simulink model "stateflow_reuseVariable"  (R2016b)
settings: Solver=VariableStepAuto  StartTime=0.0  StopTime=10.0  RelTol=1e-3  EnableMultiTasking=on
settings Model: Creator=amyyang  LastModifiedBy=amyyang
settings DataIOCC: LimitDataPoints=on
settings OptimizationCC: LifeSpan=inf
settings DebuggingCC: AllowSymbolicDim=off  SFUnexpectedBacktrackingDiag=warning  SFNoUnconditionalDefaultTransitionDiag=warning  SFExecutionAtInitializationDiag=none
settings ModelReferenceCC: PropagateSignalLabelsOutOfModel=off
settings GRTTargetCC: TargetLangStandard=C89/C90 (ANSI)
settings ConfigComp: CovMetricSettings=dw  CovHtmlReporting=on  CovSaveCumulativeToWorkspaceVar=on  CovSaveSingleToWorkspaceVar=on  CovExternalEMLEnable=off

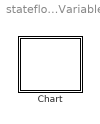
== system stateflow_reuseVariable ==
  Chart : Stateflow chart  TreatAsAtomicUnit=on

== stateflow chart stateflow_reuseVariable/Chart ==
  state A
    note: 作为循环计数器的变量，在同一个状态内，就只做这一个用途。
    (default) -> (junction 52) [order 2] : {
        |  i = 1;
        | }
    (default) -> (junction 2) [order 1] : {
        |  i = 1;
        | }
    (junction 2) -> (junction 36) [order 1] : [ i<10]
    (junction 52) -> (junction 53) [order 1] : [ i<10]
    (junction 36) -> (junction 38)
    (junction 53) -> (junction 54)
    (junction 38) -> (junction 2) : {
        |  i++;
        | }
    (junction 54) -> (junction 52) : {
        |  i++;
        | }
    (junction 2) -> (junction 40) [order 2] : {
        | c = b + a;
        | }
    (junction 52) -> (junction 49) [order 2] : {
        | i = b + a;
        | }
  state SA1
    en:
    pre1 = 0;
    pre2 = 0;
    du:
    a = alp * Tin ;
  state SA2
    en:
    a = pre2 - pre1;
  note: 这里的 a 作为各个state定义的Lcoal变量，需要在各自的state里单独定义
  (default) -> SA1
  SA1 -> SA2 : [ (engSpd < 10) || (engSpd > 9000)]
  SA2 -> SA1 : [ falg ]
